simulink model "SPGF_FSK_0000_R2022b"  (R2022b)
settings: Solver=ode4  StartTime=0.0  StopTime=1.4  FixedStep=50e-6/50  RelTol=1e-3  EnableMultiTasking=on
undefined symbols (not defined in the file): D11, Delta
libraries: spsSeriesRLCBranchLib x1646, spsGroundLib x360, spsStairGeneratorLib x147, spsIdealSwitchLib x145, spsCurrentMeasurementLib x145, spsUniversalBridgeLib x76, spsThreePhaseSeriesRLCLoadLib x57, simulink x45, spsBistableLib x36, spsSequenceAnalyzerLib x31, spsThreePhaseParallelRLCLoadLib x20, spsThreePhaseTransformerTwoWindingsLib x20
(part 34 of 40)

== system SPGF_FSK_0000_R2022b/W60/Pi ==
  Ground{,1..8} (9 alike) : spsGroundLib/Ground  LConnTagsString=a
  Series RLC Branch{,1..2,27..28,33} (6 alike) : spsSeriesRLCBranchLib/Series RLC Branch  LConnTagsString=__new0  RConnTagsString=__new0  BranchType=RL  Resistance=R/2  Inductance=L/2  SetiL0=off  InitialCurrent=0  Capacitance=1e-6  Setx0=off  InitialVoltage=0  Measurements=None
  Series RLC Branch{10..11,13,29..30,32} (6 alike) : spsSeriesRLCBranchLib/Series RLC Branch  LConnTagsString=__new0  RConnTagsString=__new0  BranchType=R  Resistance=Rfg*4  Inductance=L/2  SetiL0=off  InitialCurrent=0  Capacitance=1e-6  Setx0=off  InitialVoltage=0  Measurements=None
  Series RLC Branch{9,12,14,31,40..41} (6 alike) : spsSeriesRLCBranchLib/Series RLC Branch  LConnTagsString=__new0  RConnTagsString=__new0  BranchType=C  Resistance=R/2  Inductance=L/2  SetiL0=off  InitialCurrent=0  Capacitance=Cfg*0.25  Setx0=off  InitialVoltage=0  Measurements=None
  Series RLC Branch15 : spsSeriesRLCBranchLib/Series RLC Branch  LConnTagsString=__new0  RConnTagsString=__new0  BranchType=R  Resistance=Rfg*2  Inductance=L/2  SetiL0=off  InitialCurrent=0  Capacitance=1e-6  Setx0=off  InitialVoltage=0  Measurements=None
  Series RLC Branch16 : spsSeriesRLCBranchLib/Series RLC Branch  LConnTagsString=__new0  RConnTagsString=__new0  BranchType=R  Resistance=Rfg*2  Inductance=L/2  SetiL0=off  InitialCurrent=0  Capacitance=1e-6  Setx0=off  InitialVoltage=0  Measurements=None
  Series RLC Branch17 : spsSeriesRLCBranchLib/Series RLC Branch  LConnTagsString=__new0  RConnTagsString=__new0  BranchType=C  Resistance=R/2  Inductance=L/2  SetiL0=off  InitialCurrent=0  Capacitance=Cfg*0.5  Setx0=off  InitialVoltage=0  Measurements=None
  Series RLC Branch18 : spsSeriesRLCBranchLib/Series RLC Branch  LConnTagsString=__new0  RConnTagsString=__new0  BranchType=R  Resistance=Rfg*2  Inductance=L/2  SetiL0=off  InitialCurrent=0  Capacitance=1e-6  Setx0=off  InitialVoltage=0  Measurements=None
  Series RLC Branch19 : spsSeriesRLCBranchLib/Series RLC Branch  LConnTagsString=__new0  RConnTagsString=__new0  BranchType=C  Resistance=R/2  Inductance=L/2  SetiL0=off  InitialCurrent=0  Capacitance=Cfg*0.5  Setx0=off  InitialVoltage=0  Measurements=None
  Series RLC Branch20 : spsSeriesRLCBranchLib/Series RLC Branch  LConnTagsString=__new0  RConnTagsString=__new0  BranchType=C  Resistance=R/2  Inductance=L/2  SetiL0=off  InitialCurrent=0  Capacitance=Cmf*0.5  Setx0=off  InitialVoltage=0  Measurements=None
  Series RLC Branch21 : spsSeriesRLCBranchLib/Series RLC Branch  LConnTagsString=__new0  RConnTagsString=__new0  BranchType=R  Resistance=Rmf*2  Inductance=L/2  SetiL0=off  InitialCurrent=0  Capacitance=1e-6  Setx0=off  InitialVoltage=0  Measurements=None
  Series RLC Branch22 : spsSeriesRLCBranchLib/Series RLC Branch  LConnTagsString=__new0  RConnTagsString=__new0  BranchType=C  Resistance=R/2  Inductance=L/2  SetiL0=off  InitialCurrent=0  Capacitance=Cmf*0.5  Setx0=off  InitialVoltage=0  Measurements=None
  Series RLC Branch23 : spsSeriesRLCBranchLib/Series RLC Branch  LConnTagsString=__new0  RConnTagsString=__new0  BranchType=R  Resistance=Rmf*2  Inductance=L/2  SetiL0=off  InitialCurrent=0  Capacitance=1e-6  Setx0=off  InitialVoltage=0  Measurements=None
  Series RLC Branch24 : spsSeriesRLCBranchLib/Series RLC Branch  LConnTagsString=__new0  RConnTagsString=__new0  BranchType=C  Resistance=R/2  Inductance=L/2  SetiL0=off  InitialCurrent=0  Capacitance=Cmf*0.5  Setx0=off  InitialVoltage=0  Measurements=None
  Series RLC Branch25 : spsSeriesRLCBranchLib/Series RLC Branch  LConnTagsString=__new0  RConnTagsString=__new0  BranchType=R  Resistance=Rmf*2  Inductance=L/2  SetiL0=off  InitialCurrent=0  Capacitance=1e-6  Setx0=off  InitialVoltage=0  Measurements=None
  Series RLC Branch26 : spsSeriesRLCBranchLib/Series RLC Branch  LConnTagsString=__new0  RConnTagsString=__new0  BranchType=C  Resistance=R/2  Inductance=L/2  SetiL0=off  InitialCurrent=0  Capacitance=Cfg*0.5  Setx0=off  InitialVoltage=0  Measurements=None
  Series RLC Branch{3,5,7,34,36,38} (6 alike) : spsSeriesRLCBranchLib/Series RLC Branch  LConnTagsString=__new0  RConnTagsString=__new0  BranchType=C  Resistance=R/2  Inductance=L/2  SetiL0=off  InitialCurrent=0  Capacitance=Cmf*0.25  Setx0=off  InitialVoltage=0  Measurements=None
  Series RLC Branch{4,6,8,35,37,39} (6 alike) : spsSeriesRLCBranchLib/Series RLC Branch  LConnTagsString=__new0  RConnTagsString=__new0  BranchType=R  Resistance=Rmf*4  Inductance=L/2  SetiL0=off  InitialCurrent=0  Capacitance=1e-6  Setx0=off  InitialVoltage=0  Measurements=None
  A : PMIOPort  Side=Left
  B : PMIOPort  Port=2  Side=Left
  C : PMIOPort  Port=3  Side=Left
  a : PMIOPort  Port=4  Side=Right
  b : PMIOPort  Port=5  Side=Right
  c : PMIOPort  Port=6  Side=Right
  connections:
  Series RLC Branch12/LConn1 -- Series RLC Branch11/LConn1 -- Series RLC Branch5/LConn1 -- Series RLC Branch6/LConn1 -- B/RConn1 -- Series RLC Branch4/RConn1 -- Series RLC Branch3/RConn1 -- Series RLC Branch1/LConn1
  Series RLC Branch13/LConn1 -- A/RConn1 -- Series RLC Branch4/LConn1 -- Series RLC Branch3/LConn1 -- Series RLC Branch7/LConn1 -- Series RLC Branch8/LConn1 -- Series RLC Branch/LConn1 -- Series RLC Branch14/LConn1
  Series RLC Branch9/LConn1 -- Series RLC Branch2/LConn1 -- Series RLC Branch8/RConn1 -- Series RLC Branch7/RConn1 -- C/RConn1 -- Series RLC Branch5/RConn1 -- Series RLC Branch6/RConn1 -- Series RLC Branch10/LConn1
  Series RLC Branch9/RConn1 -- Ground/LConn1 -- Series RLC Branch10/RConn1
  Series RLC Branch12/RConn1 -- Series RLC Branch11/RConn1 -- Ground1/LConn1
  Series RLC Branch13/RConn1 -- Series RLC Branch14/RConn1 -- Ground2/LConn1
  Series RLC Branch17/LConn1 -- Series RLC Branch16/LConn1 -- Series RLC Branch28/LConn1 -- Series RLC Branch1/RConn1 -- Series RLC Branch23/LConn1 -- Series RLC Branch22/LConn1 -- Series RLC Branch20/RConn1 -- Series RLC Branch21/RConn1
  Series RLC Branch21/LConn1 -- Series RLC Branch20/LConn1 -- Series RLC Branch/RConn1 -- Series RLC Branch27/LConn1 -- Series RLC Branch19/LConn1 -- Series RLC Branch18/LConn1 -- Series RLC Branch24/LConn1 -- Series RLC Branch25/LConn1
  Series RLC Branch26/LConn1 -- Series RLC Branch15/LConn1 -- Series RLC Branch2/RConn1 -- Series RLC Branch33/LConn1 -- Series RLC Branch25/RConn1 -- Series RLC Branch24/RConn1 -- Series RLC Branch22/RConn1 -- Series RLC Branch23/RConn1
  Series RLC Branch26/RConn1 -- Series RLC Branch15/RConn1 -- Ground3/LConn1
  Ground4/LConn1 -- Series RLC Branch17/RConn1 -- Series RLC Branch16/RConn1
  Ground5/LConn1 -- Series RLC Branch18/RConn1 -- Series RLC Branch19/RConn1
  Series RLC Branch31/LConn1 -- b/RConn1 -- Series RLC Branch35/RConn1 -- Series RLC Branch34/RConn1 -- Series RLC Branch36/LConn1 -- Series RLC Branch37/LConn1 -- Series RLC Branch28/RConn1 -- Series RLC Branch30/LConn1
  Series RLC Branch34/LConn1 -- a/RConn1 -- Series RLC Branch41/LConn1 -- Series RLC Branch32/LConn1 -- Series RLC Branch38/LConn1 -- Series RLC Branch39/LConn1 -- Series RLC Branch27/RConn1 -- Series RLC Branch35/LConn1
  Series RLC Branch29/LConn1 -- Series RLC Branch36/RConn1 -- Series RLC Branch37/RConn1 -- c/RConn1 -- Series RLC Branch39/RConn1 -- Series RLC Branch38/RConn1 -- Series RLC Branch33/RConn1 -- Series RLC Branch40/LConn1
  Series RLC Branch29/RConn1 -- Series RLC Branch40/RConn1 -- Ground6/LConn1
  Series RLC Branch31/RConn1 -- Series RLC Branch30/RConn1 -- Ground7/LConn1
  Series RLC Branch32/RConn1 -- Series RLC Branch41/RConn1 -- Ground8/LConn1

== system SPGF_FSK_0000_R2022b/W60/Q ==
  breaker : Subsystem  Commented=on  mask{SwitchA=off, SwitchB=off, SwitchC=off, InitialStatus=[1 1 1], BreakerResistance=0.0001, SnubberResistance=1e6, SnubberCapacitance=inf, TransitionTimes=[0.5 0.7], ShiftTimes=[0 0 0]}
      mask prompts: SwitchA "Switching of phase A"; SwitchB "Switching of phase B"; SwitchC "Switching of phase C"; InitialStatus "Initial status of phase breaker [A, B, C]"; BreakerResistance "Breaker resistance Ron (ohms) :"; SnubberResistance "Snubbers resistance Rp (ohms) :"; SnubberCapacitance "Snubbers capacitance Cp (F) :"; TransitionTimes "Transition times (s) :"; ShiftTimes "Time differences for switch [tA, tB, tC] (s) :"
      mask init: same as SPGF_FSK_0000_R2022b/Feed/Q/breaker
      mask Display:
      | % port_label('input',1,'Iabc');
      | 
      | port_label('lconn',1,'A');
      | port_label('lconn',2,'B');
      | port_label('lconn',3,'C');
      | 
      | port_label('rconn',1,'a');
      | port_label('rconn',2,'b');
      | port_label('rconn',3,'c');
      | 
      | disp('   Q    ');
  meas : Subsystem
  shunt : Subsystem
  A : PMIOPort  Side=Right
  B : PMIOPort  Port=2  Side=Right
  C : PMIOPort  Port=3  Side=Right
  a : PMIOPort  Port=4  Side=Left
  b : PMIOPort  Port=5  Side=Left
  c : PMIOPort  Port=6  Side=Left
  connections:
  shunt/LConn3 -- C/RConn1 -- breaker/LConn3
  shunt/LConn2 -- B/RConn1 -- breaker/LConn2
  A/RConn1 -- shunt/LConn1 -- breaker/LConn1
  meas/RConn1 -- a/RConn1
  meas/RConn2 -- b/RConn1
  meas/RConn3 -- c/RConn1
  meas/LConn3 -- breaker/RConn3 -- shunt/RConn3
  meas/LConn2 -- breaker/RConn2 -- shunt/RConn2
  meas/LConn1 -- breaker/RConn1 -- shunt/RConn1

== system SPGF_FSK_0000_R2022b/W60/concentrated ==
  Ccs/1 : spsSeriesRLCBranchLib/Series RLC Branch  LConnTagsString=__new0  RConnTagsString=__new0  BranchType=C  Resistance=190  Inductance=1e-3  SetiL0=off  InitialCurrent=0  Capacitance=-C_matrix(1,2)/2  Setx0=off  InitialVoltage=0  Measurements=None
  Ccs/2 : spsSeriesRLCBranchLib/Series RLC Branch  LConnTagsString=__new0  RConnTagsString=__new0  BranchType=C  Resistance=190  Inductance=1e-3  SetiL0=off  InitialCurrent=0  Capacitance=-C_matrix(1,2)/2  Setx0=off  InitialVoltage=0  Measurements=None
  Ccs2/1 : spsSeriesRLCBranchLib/Series RLC Branch  LConnTagsString=__new0  RConnTagsString=__new0  BranchType=C  Resistance=190  Inductance=1e-3  SetiL0=off  InitialCurrent=0  Capacitance=-C_matrix(3,4)/2  Setx0=off  InitialVoltage=0  Measurements=None
  Ccs2/2 : spsSeriesRLCBranchLib/Series RLC Branch  LConnTagsString=__new0  RConnTagsString=__new0  BranchType=C  Resistance=190  Inductance=1e-3  SetiL0=off  InitialCurrent=0  Capacitance=-C_matrix(3,4)/2  Setx0=off  InitialVoltage=0  Measurements=None
  Ccs2/3 : spsSeriesRLCBranchLib/Series RLC Branch  LConnTagsString=__new0  RConnTagsString=__new0  BranchType=R  Resistance=-Rg_matrix(3,4)*2  Inductance=1e-3  SetiL0=off  InitialCurrent=0  Capacitance=Rg_matrix(3,4)*2  Setx0=off  InitialVoltage=0  Measurements=None
  Ccs2/4 : spsSeriesRLCBranchLib/Series RLC Branch  LConnTagsString=__new0  RConnTagsString=__new0  BranchType=R  Resistance=-Rg_matrix(3,4)*2  Inductance=1e-3  SetiL0=off  InitialCurrent=0  Capacitance=Rg_matrix(3,4)*2  Setx0=off  InitialVoltage=0  Measurements=None
  Ccs3/1 : spsSeriesRLCBranchLib/Series RLC Branch  LConnTagsString=__new0  RConnTagsString=__new0  BranchType=C  Resistance=190  Inductance=1e-3  SetiL0=off  InitialCurrent=0  Capacitance=-C_matrix(5,6)/2  Setx0=off  InitialVoltage=0  Measurements=None
  Ccs3/2 : spsSeriesRLCBranchLib/Series RLC Branch  LConnTagsString=__new0  RConnTagsString=__new0  BranchType=C  Resistance=190  Inductance=1e-3  SetiL0=off  InitialCurrent=0  Capacitance=-C_matrix(5,6)/2  Setx0=off  InitialVoltage=0  Measurements=None
  Ccs3/3 : spsSeriesRLCBranchLib/Series RLC Branch  LConnTagsString=__new0  RConnTagsString=__new0  BranchType=R  Resistance=-Rg_matrix(5,6)*2  Inductance=1e-3  SetiL0=off  InitialCurrent=0  Capacitance=-C_matrix(5,6)/2  Setx0=off  InitialVoltage=0  Measurements=None
  Ccs3/4 : spsSeriesRLCBranchLib/Series RLC Branch  LConnTagsString=__new0  RConnTagsString=__new0  BranchType=R  Resistance=-Rg_matrix(5,6)*2  Inductance=1e-3  SetiL0=off  InitialCurrent=0  Capacitance=-C_matrix(5,6)/2  Setx0=off  InitialVoltage=0  Measurements=None
  Csg/2 : spsSeriesRLCBranchLib/Series RLC Branch  LConnTagsString=__new0  RConnTagsString=__new0  BranchType=C  Resistance=190  Inductance=1e-3  SetiL0=off  InitialCurrent=0  Capacitance=( C_matrix(1,2) + C_matrix(2,2) )/2  Setx0=off  InitialVoltage=0  Measurements=None
  Csg1/1 : spsSeriesRLCBranchLib/Series RLC Branch  LConnTagsString=__new0  RConnTagsString=__new0  BranchType=C  Resistance=190  Inductance=1e-3  SetiL0=off  InitialCurrent=0  Capacitance=( C_matrix(1,2) + C_matrix(2,2) )/2  Setx0=off  InitialVoltage=0  Measurements=None
  Csg2/1 : spsSeriesRLCBranchLib/Series RLC Branch  LConnTagsString=__new0  RConnTagsString=__new0  BranchType=C  Resistance=190  Inductance=1e-3  SetiL0=off  InitialCurrent=0  Capacitance=( C_matrix(3,4) + C_matrix(4,4) )/2  Setx0=off  InitialVoltage=0  Measurements=None
  Csg2/2 : spsSeriesRLCBranchLib/Series RLC Branch  LConnTagsString=__new0  RConnTagsString=__new0  BranchType=C  Resistance=190  Inductance=1e-3  SetiL0=off  InitialCurrent=0  Capacitance=( C_matrix(3,4) + C_matrix(4,4) )/2  Setx0=off  InitialVoltage=0  Measurements=None
  Csg3/1 : spsSeriesRLCBranchLib/Series RLC Branch  LConnTagsString=__new0  RConnTagsString=__new0  BranchType=C  Resistance=190  Inductance=1e-3  SetiL0=off  InitialCurrent=0  Capacitance=( C_matrix(5,6) + C_matrix(6,6) ) /2  Setx0=off  InitialVoltage=0  Measurements=None
  Csg3/2 : spsSeriesRLCBranchLib/Series RLC Branch  LConnTagsString=__new0  RConnTagsString=__new0  BranchType=C  Resistance=190  Inductance=1e-3  SetiL0=off  InitialCurrent=0  Capacitance=( C_matrix(5,6) + C_matrix(6,6) ) /2  Setx0=off  InitialVoltage=0  Measurements=None
  Ground{1..4} (4 alike) : spsGroundLib/Ground  LConnTagsString=a
  RL : spsMutualInductanceLib/Mutual Inductance  LConnTagsString=a|b|c|L4|L5|L6  RConnTagsString=A|B|C|R4|R5|R6  TypeOfMutual=Generalized mutual inductance  NumberOfWindings=6  SelfImpedance1=[1.1 1.1e-03]  SelfImpedance2=[ 1.1 1.1e-03]  ThreeWindings=on  SelfImpedance3=[ 1.1 1.1e-03]  MutualImpedance=[1.0 1.0e-03]  InductanceMatrix=L_matrix  ResistanceMatrix=R_matrix  Measurements=None
      settings: LibrarySourceBlock=sps_lib/Passives/Mutual Inductance
  Rcs*2 : spsSeriesRLCBranchLib/Series RLC Branch  LConnTagsString=__new0  RConnTagsString=__new0  BranchType=R  Resistance=-Rg_matrix(1,2)*2  Inductance=1e-3  SetiL0=off  InitialCurrent=0  Capacitance=Rg_matrix(1,2)*2  Setx0=off  InitialVoltage=0  Measurements=None
  Rgcs1/1 : spsSeriesRLCBranchLib/Series RLC Branch  LConnTagsString=__new0  RConnTagsString=__new0  BranchType=R  Resistance=-Rg_matrix(1,2)*2  Inductance=1e-3  SetiL0=off  InitialCurrent=0  Capacitance=Rg_matrix(1,2)*2  Setx0=off  InitialVoltage=0  Measurements=None
  Rgsg1/1 : spsSeriesRLCBranchLib/Series RLC Branch  LConnTagsString=__new0  RConnTagsString=__new0  BranchType=R  Resistance=(Rg_matrix(4,4)+Rg_matrix(3,4))*2  Inductance=1e-3  SetiL0=off  InitialCurrent=0  Capacitance=Rg_matrix(1,2)*2  Setx0=off  InitialVoltage=0  Measurements=None
  Rgsg1/2 : spsSeriesRLCBranchLib/Series RLC Branch  LConnTagsString=__new0  RConnTagsString=__new0  BranchType=R  Resistance=(Rg_matrix(2,2)+Rg_matrix(1,2))*2  Inductance=1e-3  SetiL0=off  InitialCurrent=0  Capacitance=Rg_matrix(1,2)*2  Setx0=off  InitialVoltage=0  Measurements=None
  Rgsg1/3 : spsSeriesRLCBranchLib/Series RLC Branch  LConnTagsString=__new0  RConnTagsString=__new0  BranchType=R  Resistance=(Rg_matrix(4,4)+Rg_matrix(3,4))*2  Inductance=1e-3  SetiL0=off  InitialCurrent=0  Capacitance=Rg_matrix(1,2)*2  Setx0=off  InitialVoltage=0  Measurements=None
  Rgsg1/4 : spsSeriesRLCBranchLib/Series RLC Branch  LConnTagsString=__new0  RConnTagsString=__new0  BranchType=R  Resistance=(Rg_matrix(2,2)+Rg_matrix(1,2))*2  Inductance=1e-3  SetiL0=off  InitialCurrent=0  Capacitance=Rg_matrix(1,2)*2  Setx0=off  InitialVoltage=0  Measurements=None
  Rsg*2 : spsSeriesRLCBranchLib/Series RLC Branch  LConnTagsString=__new0  RConnTagsString=__new0  BranchType=R  Resistance=(Rg_matrix(6,6)+Rg_matrix(5,6))*2  Inductance=1e-3  SetiL0=off  InitialCurrent=0  Capacitance=Rg_matrix(1,2)*2  Setx0=off  InitialVoltage=0  Measurements=None
  Rsg1/1 : spsSeriesRLCBranchLib/Series RLC Branch  LConnTagsString=__new0  RConnTagsString=__new0  BranchType=R  Resistance=(Rg_matrix(6,6)+Rg_matrix(5,6))*2  Inductance=1e-3  SetiL0=off  InitialCurrent=0  Capacitance=Rg_matrix(1,2)*2  Setx0=off  InitialVoltage=0  Measurements=None
  A : PMIOPort  Side=Left
  B : PMIOPort  Port=2  Side=Left
  C : PMIOPort  Port=3  Side=Left
  a : PMIOPort  Port=4  Side=Right
  b : PMIOPort  Port=5  Side=Right
  c : PMIOPort  Port=6  Side=Right
  connections:
  RL/LConn6 -- Ground3/LConn1 -- Rgsg1/2/LConn1 -- Csg/2/LConn1 -- Rcs*2/LConn1 -- Ccs/2/LConn1 -- RL/LConn2 -- RL/LConn4 -- Rgsg1/1/LConn1 -- Csg2/2/LConn1 -- Ccs2/3/LConn1 -- Ccs2/2/LConn1 -- Rsg*2/LConn1 -- Csg3/2/LConn1 -- Ccs3/3/LConn1 -- Ccs3/2/LConn1
  Rsg1/1/RConn1 -- Rgsg1/3/RConn1 -- Rgsg1/4/RConn1 -- Csg3/1/RConn1 -- Csg2/1/RConn1 -- Ground2/LConn1 -- Csg1/1/RConn1
  Rgsg1/3/LConn1 -- Ccs2/4/LConn1 -- Csg2/1/LConn1 -- Ccs2/1/LConn1 -- RL/RConn4 -- Rgsg1/4/LConn1 -- Rgcs1/1/LConn1 -- Csg1/1/LConn1 -- Ccs/1/LConn1 -- RL/RConn2 -- Ground4/LConn1 -- RL/RConn6 -- Ccs3/1/LConn1 -- Rsg1/1/LConn1 -- Ccs3/4/LConn1 -- Csg3/1/LConn1
  Rsg*2/RConn1 -- Rgsg1/1/RConn1 -- Rgsg1/2/RConn1 -- Csg3/2/RConn1 -- Csg2/2/RConn1 -- Ground1/LConn1 -- Csg/2/RConn1
  a/RConn1 -- RL/RConn1 -- Rgcs1/1/RConn1 -- Ccs/1/RConn1
  b/RConn1 -- RL/RConn3 -- Ccs2/4/RConn1 -- Ccs2/1/RConn1
  Ccs3/1/RConn1 -- c/RConn1 -- RL/RConn5 -- Ccs3/4/RConn1
  RL/LConn1 -- A/RConn1 -- Rcs*2/RConn1 -- Ccs/2/RConn1
  RL/LConn3 -- B/RConn1 -- Ccs2/3/RConn1 -- Ccs2/2/RConn1
  Ccs3/2/RConn1 -- C/RConn1 -- RL/LConn5 -- Ccs3/3/RConn1

== system SPGF_FSK_0000_R2022b/W61/Q ==
  breaker : Subsystem  Commented=on  mask{SwitchA=off, SwitchB=off, SwitchC=off, InitialStatus=[1 1 1], BreakerResistance=0.0001, SnubberResistance=1e6, SnubberCapacitance=inf, TransitionTimes=[0.5 0.7], ShiftTimes=[0 0 0]}
      mask prompts: SwitchA "Switching of phase A"; SwitchB "Switching of phase B"; SwitchC "Switching of phase C"; InitialStatus "Initial status of phase breaker [A, B, C]"; BreakerResistance "Breaker resistance Ron (ohms) :"; SnubberResistance "Snubbers resistance Rp (ohms) :"; SnubberCapacitance "Snubbers capacitance Cp (F) :"; TransitionTimes "Transition times (s) :"; ShiftTimes "Time differences for switch [tA, tB, tC] (s) :"
      mask init: same as SPGF_FSK_0000_R2022b/Feed/Q/breaker
      mask Display:
      | % port_label('input',1,'Iabc');
      | 
      | port_label('lconn',1,'A');
      | port_label('lconn',2,'B');
      | port_label('lconn',3,'C');
      | 
      | port_label('rconn',1,'a');
      | port_label('rconn',2,'b');
      | port_label('rconn',3,'c');
      | 
      | disp('   Q    ');
  meas : Subsystem
  shunt : Subsystem
  A : PMIOPort  Side=Right
  B : PMIOPort  Port=2  Side=Right
  C : PMIOPort  Port=3  Side=Right
  a : PMIOPort  Port=4  Side=Left
  b : PMIOPort  Port=5  Side=Left
  c : PMIOPort  Port=6  Side=Left
  connections:
  shunt/RConn1 -- breaker/RConn1 -- meas/LConn1
  shunt/RConn2 -- breaker/RConn2 -- meas/LConn2
  shunt/RConn3 -- breaker/RConn3 -- meas/LConn3
  meas/RConn3 -- c/RConn1
  meas/RConn2 -- b/RConn1
  meas/RConn1 -- a/RConn1
  breaker/LConn1 -- shunt/LConn1 -- A/RConn1
  breaker/LConn2 -- B/RConn1 -- shunt/LConn2
  breaker/LConn3 -- C/RConn1 -- shunt/LConn3

== system SPGF_FSK_0000_R2022b/measurements/Fourier Block abc ==
  abc : Inport
  Demux1 : Demux  Commented=on  Outputs=9
  Scope13 : Scope
  Sequence Analyzer9 : spsSequenceAnalyzerLib/Sequence Analyzer  Freq=50  n=17  seq=Positive  InInit=[0, 0]  Ts=FTime
      settings: LibrarySourceBlock=sps_lib/Sensors and Measurements/Sequence Analyzer
  Terminator9 : Terminator
  wires:
  abc/1 -> Sequence Analyzer9/1
  Sequence Analyzer9/2 -> Terminator9/1
  Sequence Analyzer9/1 -> Scope13/1, Demux1/1

== system SPGF_FSK_0000_R2022b/measurements/Fourier Block u ==
  u : Inport
  Demux1 : Demux  Commented=on  Outputs=9
  Fourier10 : spsFourierLib/Fourier  Freq=50  n=[1 2 3 5 7 9 11 13 17]  InInit=[0, 0]  Ts=FTime
  Scope13 : Scope
  Terminator10 : Terminator
  wires:
  u/1 -> Fourier10/1
  Fourier10/1 -> Demux1/1, Scope13/1
  Fourier10/2 -> Terminator10/1

== system SPGF_FSK_0000_R2022b/measurements/PQ1 ==
  Vmag_seq : Inport
  Vang : Inport  Port=2
  Imag_seq : Inport  Port=3
  Iang : Inport  Port=4
  Deg->Rad : Gain  Gain=pi/180  SaturateOnIntegerOverflow=on  OutDataTypeStr=Inherit: Same as input  ParamDataTypeStr=Inherit: Same as input
  Gain1 : Gain  Gain=3/2  SaturateOnIntegerOverflow=on  OutDataTypeStr=Inherit: Same as input  ParamDataTypeStr=Inherit: Same as input
  Product : Product  InputSameDT=on  SaturateOnIntegerOverflow=on  OutDataTypeStr=Inherit: Same as first input
  Product1 : Product  InputSameDT=on  SaturateOnIntegerOverflow=on  OutDataTypeStr=Inherit: Same as first input
  Product3 : Product  InputSameDT=on  SaturateOnIntegerOverflow=on  OutDataTypeStr=Inherit: Same as first input
  Sum : Sum  Inputs=+-  InputSameDT=on  SaturateOnIntegerOverflow=on  OutDataTypeStr=Inherit: Same as first input
  Trigonometric Function1 : Trigonometry  Operator=cos
  Trigonometric Function2 : Trigonometry
  P : Outport
  Q : Outport  Port=2
  wires:
  Trigonometric Function1/1 -> Product1/2
  Sum/1 -> Deg->Rad/1
  Imag_seq/1 -> Product/2
  Product/1 -> Gain1/1  "V1 *I1"
  Trigonometric Function2/1 -> Product3/2
  Gain1/1 -> Product1/1, Product3/1
  Vmag_seq/1 -> Product/1
  Deg->Rad/1 -> Trigonometric Function2/1, Trigonometric Function1/1  "phi"
  Product3/1 -> Q/1
  Iang/1 -> Sum/2
  Vang/1 -> Sum/1
  Product1/1 -> P/1

== system SPGF_FSK_0000_R2022b/measurements/PQ8 ==
  Vmag_seq : Inport
  Vang : Inport  Port=2
  Imag_seq : Inport  Port=3
  Iang : Inport  Port=4
  Deg->Rad : Gain  Gain=pi/180  SaturateOnIntegerOverflow=on  OutDataTypeStr=Inherit: Same as input  ParamDataTypeStr=Inherit: Same as input
  Gain1 : Gain  Gain=3/2  SaturateOnIntegerOverflow=on  OutDataTypeStr=Inherit: Same as input  ParamDataTypeStr=Inherit: Same as input
  Product : Product  InputSameDT=on  SaturateOnIntegerOverflow=on  OutDataTypeStr=Inherit: Same as first input
  Product1 : Product  InputSameDT=on  SaturateOnIntegerOverflow=on  OutDataTypeStr=Inherit: Same as first input
  Product3 : Product  InputSameDT=on  SaturateOnIntegerOverflow=on  OutDataTypeStr=Inherit: Same as first input
  Sum : Sum  Inputs=+-  InputSameDT=on  SaturateOnIntegerOverflow=on  OutDataTypeStr=Inherit: Same as first input
  Trigonometric Function1 : Trigonometry  Operator=cos
  Trigonometric Function2 : Trigonometry
  P : Outport
  Q : Outport  Port=2
  wires:
  Product1/1 -> P/1
  Vang/1 -> Sum/1
  Iang/1 -> Sum/2
  Product3/1 -> Q/1
  Deg->Rad/1 -> Trigonometric Function1/1, Trigonometric Function2/1  "phi"
  Vmag_seq/1 -> Product/1
  Gain1/1 -> Product3/1, Product1/1
  Trigonometric Function2/1 -> Product3/2
  Product/1 -> Gain1/1  "V1 *I1"
  Imag_seq/1 -> Product/2
  Sum/1 -> Deg->Rad/1
  Trigonometric Function1/1 -> Product1/2

== system SPGF_FSK_0000_R2022b/measurements/RMS1 ==
  abc : Inport
  Gain25 : Gain  Gain=1/sqrt(2)
  Rate Transition : RateTransition
  Rate Transition1 : RateTransition
  Sequence Analyzer : spsSequenceAnalyzerLib/Sequence Analyzer  Freq=50  n=1  seq=Positive  InInit=[1, 0]  Ts=FTime
      settings: LibrarySourceBlock=sps_lib/Sensors and Measurements/Sequence Analyzer
  Terminator19 : Terminator
  I1 : Outport
  wires:
  Sequence Analyzer/2 -> Terminator19/1
  Gain25/1 -> Rate Transition1/1
  Sequence Analyzer/1 -> Gain25/1
  abc/1 -> Rate Transition/1
  Rate Transition/1 -> Sequence Analyzer/1
  Rate Transition1/1 -> I1/1

== system SPGF_FSK_0000_R2022b/measurements/RMS10 ==
  i : Inport
  Fourier36 : spsFourierLib/Fourier  Freq=50  n=1  InInit=[0, 0]  Ts=FTime
  Gain25 : Gain  Gain=1/sqrt(2)
  Rate Transition : RateTransition
  Rate Transition1 : RateTransition
  Terminator19 : Terminator
  I : Outport
  wires:
  Rate Transition1/1 -> I/1
  Rate Transition/1 -> Fourier36/1
  Fourier36/2 -> Terminator19/1
  Gain25/1 -> Rate Transition1/1
  Fourier36/1 -> Gain25/1
  i/1 -> Rate Transition/1

== system SPGF_FSK_0000_R2022b/measurements/RMS11 ==
  i : Inport
  Fourier36 : spsFourierLib/Fourier  Freq=50  n=1  InInit=[0, 0]  Ts=FTime
  Gain25 : Gain  Gain=1/sqrt(2)
  Rate Transition : RateTransition
  Rate Transition1 : RateTransition
  Terminator19 : Terminator
  I : Outport
  wires:
  i/1 -> Rate Transition/1
  Fourier36/1 -> Gain25/1
  Gain25/1 -> Rate Transition1/1
  Fourier36/2 -> Terminator19/1
  Rate Transition/1 -> Fourier36/1
  Rate Transition1/1 -> I/1

== system SPGF_FSK_0000_R2022b/measurements/RMS12 ==
  abc : Inport
  Gain25 : Gain  Gain=1/sqrt(2)
  Rate Transition : RateTransition
  Rate Transition1 : RateTransition
  Sequence Analyzer : spsSequenceAnalyzerLib/Sequence Analyzer  Freq=50  n=1  seq=Positive  InInit=[1, 0]  Ts=FTime
      settings: LibrarySourceBlock=sps_lib/Sensors and Measurements/Sequence Analyzer
  Terminator19 : Terminator
  I1 : Outport
  wires:
  Sequence Analyzer/2 -> Terminator19/1
  Gain25/1 -> Rate Transition1/1
  Sequence Analyzer/1 -> Gain25/1
  abc/1 -> Rate Transition/1
  Rate Transition/1 -> Sequence Analyzer/1
  Rate Transition1/1 -> I1/1

== system SPGF_FSK_0000_R2022b/measurements/RMS13 ==
  i : Inport
  Fourier36 : spsFourierLib/Fourier  Freq=50  n=1  InInit=[0, 0]  Ts=FTime
  Gain25 : Gain  Gain=1/sqrt(2)
  Rate Transition : RateTransition
  Rate Transition1 : RateTransition
  Terminator19 : Terminator
  I : Outport
  wires:
  Rate Transition1/1 -> I/1
  Rate Transition/1 -> Fourier36/1
  Fourier36/2 -> Terminator19/1
  Gain25/1 -> Rate Transition1/1
  Fourier36/1 -> Gain25/1
  i/1 -> Rate Transition/1

== system SPGF_FSK_0000_R2022b/measurements/RMS14 ==
  abc : Inport
  Gain25 : Gain  Gain=1/sqrt(2)
  Rate Transition : RateTransition
  Rate Transition1 : RateTransition
  Sequence Analyzer : spsSequenceAnalyzerLib/Sequence Analyzer  Freq=50  n=1  seq=Positive  InInit=[1, 0]  Ts=FTime
      settings: LibrarySourceBlock=sps_lib/Sensors and Measurements/Sequence Analyzer
  Terminator19 : Terminator
  I1 : Outport
  wires:
  Rate Transition1/1 -> I1/1
  Rate Transition/1 -> Sequence Analyzer/1
  abc/1 -> Rate Transition/1
  Sequence Analyzer/1 -> Gain25/1
  Gain25/1 -> Rate Transition1/1
  Sequence Analyzer/2 -> Terminator19/1

== system SPGF_FSK_0000_R2022b/measurements/RMS2 ==
  i : Inport
  Fourier36 : spsFourierLib/Fourier  Freq=50  n=1  InInit=[0, 0]  Ts=FTime
  Gain25 : Gain  Gain=1/sqrt(2)
  Rate Transition : RateTransition
  Rate Transition1 : RateTransition
  Terminator19 : Terminator
  I : Outport
  wires:
  i/1 -> Rate Transition/1
  Fourier36/1 -> Gain25/1
  Gain25/1 -> Rate Transition1/1
  Fourier36/2 -> Terminator19/1
  Rate Transition/1 -> Fourier36/1
  Rate Transition1/1 -> I/1

== system SPGF_FSK_0000_R2022b/measurements/RMS3 ==
  abc : Inport
  Gain25 : Gain  Gain=1/sqrt(2)
  Rate Transition : RateTransition
  Rate Transition1 : RateTransition
  Sequence Analyzer : spsSequenceAnalyzerLib/Sequence Analyzer  Freq=50  n=1  seq=Positive  InInit=[1, 0]  Ts=FTime
      settings: LibrarySourceBlock=sps_lib/Sensors and Measurements/Sequence Analyzer
  Terminator19 : Terminator
  I1 : Outport
  wires:
  Rate Transition1/1 -> I1/1
  Rate Transition/1 -> Sequence Analyzer/1
  abc/1 -> Rate Transition/1
  Sequence Analyzer/1 -> Gain25/1
  Gain25/1 -> Rate Transition1/1
  Sequence Analyzer/2 -> Terminator19/1

== system SPGF_FSK_0000_R2022b/measurements/RMS36 ==
  abc : Inport
  Gain25 : Gain  Gain=1/sqrt(2)
  Sequence Analyzer : spsSequenceAnalyzerLib/Sequence Analyzer  Freq=50  n=1  seq=Positive  InInit=[1, 0]  Ts=FTime
      settings: LibrarySourceBlock=sps_lib/Sensors and Measurements/Sequence Analyzer
  Terminator19 : Terminator
  I1 : Outport
  wires:
  abc/1 -> Sequence Analyzer/1
  Sequence Analyzer/1 -> Gain25/1
  Gain25/1 -> I1/1
  Sequence Analyzer/2 -> Terminator19/1

== system SPGF_FSK_0000_R2022b/measurements/RMS4 ==
  i : Inport
  Fourier36 : spsFourierLib/Fourier  Freq=50  n=1  InInit=[0, 0]  Ts=FTime
  Gain25 : Gain  Gain=1/sqrt(2)
  Rate Transition : RateTransition
  Rate Transition1 : RateTransition
  Terminator19 : Terminator
  I : Outport
  wires:
  Rate Transition1/1 -> I/1
  Rate Transition/1 -> Fourier36/1
  Fourier36/2 -> Terminator19/1
  Gain25/1 -> Rate Transition1/1
  Fourier36/1 -> Gain25/1
  i/1 -> Rate Transition/1

== system SPGF_FSK_0000_R2022b/measurements/RMS44 ==
  abc : Inport
  Gain25 : Gain  Gain=1/sqrt(2)
  Sequence Analyzer : spsSequenceAnalyzerLib/Sequence Analyzer  Freq=50  n=1  seq=Positive  InInit=[1, 0]  Ts=FTime
      settings: LibrarySourceBlock=sps_lib/Sensors and Measurements/Sequence Analyzer
  Terminator19 : Terminator
  I1 : Outport
  wires:
  Sequence Analyzer/2 -> Terminator19/1
  Gain25/1 -> I1/1
  Sequence Analyzer/1 -> Gain25/1
  abc/1 -> Sequence Analyzer/1

== system SPGF_FSK_0000_R2022b/measurements/RMS45 ==
  abc : Inport
  Gain25 : Gain  Gain=1/sqrt(2)
  Sequence Analyzer : spsSequenceAnalyzerLib/Sequence Analyzer  Freq=50  n=1  seq=Positive  InInit=[1, 0]  Ts=FTime
      settings: LibrarySourceBlock=sps_lib/Sensors and Measurements/Sequence Analyzer
  Terminator19 : Terminator
  I1 : Outport
  wires:
  abc/1 -> Sequence Analyzer/1
  Sequence Analyzer/1 -> Gain25/1
  Gain25/1 -> I1/1
  Sequence Analyzer/2 -> Terminator19/1

== system SPGF_FSK_0000_R2022b/measurements/RMS46 ==
  i : Inport
  Fourier36 : spsFourierLib/Fourier  Freq=50  n=1  InInit=[0, 0]  Ts=FTime
  Gain25 : Gain  Gain=1/sqrt(2)
  Terminator19 : Terminator
  I : Outport
  wires:
  Fourier36/2 -> Terminator19/1
  Gain25/1 -> I/1
  Fourier36/1 -> Gain25/1
  i/1 -> Fourier36/1

== system SPGF_FSK_0000_R2022b/measurements/RMS5 ==
  abc : Inport
  Gain25 : Gain  Gain=1/sqrt(2)
  Rate Transition : RateTransition
  Rate Transition1 : RateTransition
  Sequence Analyzer : spsSequenceAnalyzerLib/Sequence Analyzer  Freq=50  n=1  seq=Positive  InInit=[1, 0]  Ts=FTime
      settings: LibrarySourceBlock=sps_lib/Sensors and Measurements/Sequence Analyzer
  Terminator19 : Terminator
  I1 : Outport
  wires:
  Rate Transition1/1 -> I1/1
  Rate Transition/1 -> Sequence Analyzer/1
  abc/1 -> Rate Transition/1
  Sequence Analyzer/1 -> Gain25/1
  Gain25/1 -> Rate Transition1/1
  Sequence Analyzer/2 -> Terminator19/1

== system SPGF_FSK_0000_R2022b/measurements/RMS6 ==
  i : Inport
  Fourier36 : spsFourierLib/Fourier  Freq=50  n=1  InInit=[0, 0]  Ts=FTime
  Gain25 : Gain  Gain=1/sqrt(2)
  Rate Transition : RateTransition
  Rate Transition1 : RateTransition
  Terminator19 : Terminator
  I : Outport
  wires:
  Rate Transition1/1 -> I/1
  Rate Transition/1 -> Fourier36/1
  Fourier36/2 -> Terminator19/1
  Gain25/1 -> Rate Transition1/1
  Fourier36/1 -> Gain25/1
  i/1 -> Rate Transition/1

== system SPGF_FSK_0000_R2022b/measurements/RMS7 ==
  abc : Inport
  Gain25 : Gain  Gain=1/sqrt(2)
  Rate Transition : RateTransition
  Rate Transition1 : RateTransition
  Sequence Analyzer : spsSequenceAnalyzerLib/Sequence Analyzer  Freq=50  n=1  seq=Positive  InInit=[1, 0]  Ts=FTime
      settings: LibrarySourceBlock=sps_lib/Sensors and Measurements/Sequence Analyzer
  Terminator19 : Terminator
  I1 : Outport
  wires:
  Sequence Analyzer/2 -> Terminator19/1
  Gain25/1 -> Rate Transition1/1
  Sequence Analyzer/1 -> Gain25/1
  abc/1 -> Rate Transition/1
  Rate Transition/1 -> Sequence Analyzer/1
  Rate Transition1/1 -> I1/1

== system SPGF_FSK_0000_R2022b/measurements/RMS8 ==
  i : Inport
  Fourier36 : spsFourierLib/Fourier  Freq=50  n=1  InInit=[0, 0]  Ts=FTime
  Gain25 : Gain  Gain=1/sqrt(2)
  Rate Transition : RateTransition
  Rate Transition1 : RateTransition
  Terminator19 : Terminator
  I : Outport
  wires:
  i/1 -> Rate Transition/1
  Fourier36/1 -> Gain25/1
  Gain25/1 -> Rate Transition1/1
  Fourier36/2 -> Terminator19/1
  Rate Transition/1 -> Fourier36/1
  Rate Transition1/1 -> I/1

== system SPGF_FSK_0000_R2022b/measurements/RMS9 ==
  abc : Inport
  Gain25 : Gain  Gain=1/sqrt(2)
  Rate Transition : RateTransition
  Rate Transition1 : RateTransition
  Sequence Analyzer : spsSequenceAnalyzerLib/Sequence Analyzer  Freq=50  n=1  seq=Positive  InInit=[1, 0]  Ts=FTime
      settings: LibrarySourceBlock=sps_lib/Sensors and Measurements/Sequence Analyzer
  Terminator19 : Terminator
  I1 : Outport
  wires:
  Rate Transition1/1 -> I1/1
  Rate Transition/1 -> Sequence Analyzer/1
  abc/1 -> Rate Transition/1
  Sequence Analyzer/1 -> Gain25/1
  Gain25/1 -> Rate Transition1/1
  Sequence Analyzer/2 -> Terminator19/1

== system SPGF_FSK_0000_R2022b/measurements/RXZ1 ==
  Vmag_seq : Inport
  Vang : Inport  Port=2
  Imag_seq : Inport  Port=3
  Iang : Inport  Port=4
  Add : Sum  Inputs=+-
  Divide : Product  Inputs=*/
  Gain : Gain  Gain=pi/180
  Product : Product
  Product1 : Product
  Trigonometric Function : Trigonometry
  Trigonometric Function1 : Trigonometry  Operator=cos
  R : Outport
  X : Outport  Port=2
  Z : Outport  Port=3
  Zang : Outport  Port=4
  wires:
  Iang/1 -> Add/2
  Trigonometric Function/1 -> Product1/2
  Trigonometric Function1/1 -> Product/2
  Vang/1 -> Add/1
  Divide/1 -> Z/1, Product/1, Product1/1
  Product1/1 -> X/1
  Product/1 -> R/1
  Imag_seq/1 -> Divide/2
  Vmag_seq/1 -> Divide/1
  Gain/1 -> Trigonometric Function/1, Trigonometric Function1/1
  Add/1 -> Zang/1, Gain/1

== system SPGF_FSK_0000_R2022b/measurements/RXZ7 ==
  Vmag_seq : Inport
  Vang : Inport  Port=2
  Imag_seq : Inport  Port=3
  Iang : Inport  Port=4
  Add : Sum  Inputs=+-
  Divide : Product  Inputs=*/
  Gain : Gain  Gain=pi/180
  Product : Product
  Product1 : Product
  Trigonometric Function : Trigonometry
  Trigonometric Function1 : Trigonometry  Operator=cos
  R : Outport
  X : Outport  Port=2
  Z : Outport  Port=3
  Zang : Outport  Port=4
  wires:
  Add/1 -> Gain/1, Zang/1
  Gain/1 -> Trigonometric Function1/1, Trigonometric Function/1
  Vmag_seq/1 -> Divide/1
  Imag_seq/1 -> Divide/2
  Product/1 -> R/1
  Product1/1 -> X/1
  Divide/1 -> Product1/1, Product/1, Z/1
  Vang/1 -> Add/1
  Trigonometric Function1/1 -> Product/2
  Trigonometric Function/1 -> Product1/2
  Iang/1 -> Add/2

== system SPGF_FSK_0000_R2022b/spgf/Control ==
  m : Inport
  Add : Sum  Inputs=+-
  Arcing : Subsystem  TreatAsAtomicUnit=on
  Count Limiter : Subsystem
  Ctrl : Product  Inputs=****
  Fault A2 : Constant  Value=LimitArcNum
  Fault A3 : Constant  Value=AddTimeDelay
  Fault A4 : Constant  Value=Inter
  InitialPhaseCtrl : Subsystem  TreatAsAtomicUnit=on
  Interruption : Subsystem
  One : Constant
  SW_Int : Switch  Criteria=u2 > Threshold  Threshold=0.5  SaturateOnIntegerOverflow=off  InputSameDT=off
  SW_Limit : Switch  Criteria=u2 > Threshold  Threshold=0.5  SaturateOnIntegerOverflow=off  InputSameDT=off
  SW_TD : Switch  Criteria=u2 > Threshold  Threshold=0.5  SaturateOnIntegerOverflow=off  InputSameDT=off
  Step : Step  Time=EndFaultTime  SampleTime=0
  Step1 : Step  Time=BeginFaultTime  SampleTime=0
  Time Delay : Subsystem
  g : Outport
  wires:
  Interruption/1(O) -> SW_Int/3, [Inter]
  [Inter] -> Arcing/2(Inter)
  Ctrl/1 -> Time Delay/2(Control), SW_TD/3
  InitialPhaseCtrl/1(O) -> Ctrl/3
  SW_TD/1 -> SW_Limit/3, Count Limiter/1(I)
  Step/1 -> Add/2
  Count Limiter/2(O) -> SW_Limit/1
  Fault A4/1 -> SW_Int/2
  [F] -> Arcing/Enable
  SW_Int/1 -> Ctrl/4
  [F] -> InitialPhaseCtrl/Enable
  Step1/1 -> Add/1
  m/1 -> Arcing/1(m), InitialPhaseCtrl/1(m)
  Add/1 -> [F], Ctrl/1
  Arcing/1(O) -> Ctrl/2
  Fault A2/1 -> SW_Limit/2
  Count Limiter/1(Count) -> Time Delay/1(Count)
  Time Delay/1(O) -> SW_TD/1
  Fault A3/1 -> SW_TD/2
  One/1 -> SW_Int/1
  SW_Limit/1 -> g/1

== system SPGF_FSK_0000_R2022b/Feed/Q/breaker ==
  Fault A2 : Constant  Value=InitialStatus(3)
  Fault A3 : Constant  Value=InitialStatus(2)
  Fault A4 : Constant  Value=InitialStatus(1)
  Fault C1 : Constant  Value=SwitchC
  Fault C2 : Constant  Value=SwitchB
  Fault C3 : Constant  Value=SwitchA
  Ideal Switch A : spsIdealSwitchLib/Ideal Switch  Ron=BreakerResistance  Lon=0  IC=InitialStatus(1)  Rs=SnubberResistance  Cs=SnubberCapacitance  Measurements=off
  Ideal Switch B : spsIdealSwitchLib/Ideal Switch  Ron=BreakerResistance  Lon=0  IC=InitialStatus(2)  Rs=SnubberResistance  Cs=SnubberCapacitance  Measurements=off
  Ideal Switch C : spsIdealSwitchLib/Ideal Switch  Ron=BreakerResistance  Lon=0  IC=InitialStatus(3)  Rs=SnubberResistance  Cs=SnubberCapacitance  Measurements=off
  Stair Generator A : spsStairGeneratorLib/Stair Generator  t=SwitchTimesA  e=SwitchStatusA  Ts=0
  Stair Generator B : spsStairGeneratorLib/Stair Generator  t=SwitchTimesB  e=SwitchStatusB  Ts=0
  Stair Generator C : spsStairGeneratorLib/Stair Generator  t=SwitchTimesB  e=SwitchStatusB  Ts=0
  Switch2 : Switch  Criteria=u2 > Threshold  Threshold=0.5  SaturateOnIntegerOverflow=off  InputSameDT=off
  Switch3 : Switch  Criteria=u2 > Threshold  Threshold=0.5  SaturateOnIntegerOverflow=off  InputSameDT=off
  Switch4 : Switch  Criteria=u2 > Threshold  Threshold=0.5  SaturateOnIntegerOverflow=off  InputSameDT=off
  A : PMIOPort  Side=Left
  B : PMIOPort  Port=2  Side=Left
  C : PMIOPort  Port=3  Side=Left
  a : PMIOPort  Port=4  Side=Right
  b : PMIOPort  Port=5  Side=Right
  c : PMIOPort  Port=6  Side=Right
  wires:
  Switch2/1 -> Ideal Switch C/1
  Fault A2/1 -> Switch2/3
  Fault C1/1 -> Switch2/2
  Switch3/1 -> Ideal Switch B/1
  Fault A3/1 -> Switch3/3
  Fault C2/1 -> Switch3/2
  Fault A4/1 -> Switch4/3
  Fault C3/1 -> Switch4/2
  Switch4/1 -> Ideal Switch A/1
  Stair Generator B/1 -> Switch3/1
  Stair Generator A/1 -> Switch4/1
  Stair Generator C/1 -> Switch2/1
  connections:
  Ideal Switch B/LConn1 -- B/RConn1
  Ideal Switch A/LConn1 -- A/RConn1
  Ideal Switch C/LConn1 -- C/RConn1
  Ideal Switch A/RConn1 -- a/RConn1
  b/RConn1 -- Ideal Switch B/RConn1
  c/RConn1 -- Ideal Switch C/RConn1

== system SPGF_FSK_0000_R2022b/Feed/Q/meas ==
  Add : Sum  Inputs=+++
  GainI : Gain
  GainI0 : Gain
  I A: : spsCurrentMeasurementLib/Current Measurement  PhasorSimulation=off  OutputType=Complex  PSBequivalent=0
  I B: : spsCurrentMeasurementLib/Current Measurement  PhasorSimulation=off  OutputType=Complex  PSBequivalent=0
  I C: : spsCurrentMeasurementLib/Current Measurement  PhasorSimulation=off  OutputType=Complex  PSBequivalent=0
  Mux : Mux  Inputs=3
  A : PMIOPort  Side=Left
  B : PMIOPort  Port=2  Side=Left
  C : PMIOPort  Port=3  Side=Left
  a : PMIOPort  Port=4  Side=Right
  b : PMIOPort  Port=5  Side=Right
  c : PMIOPort  Port=6  Side=Right
  tag scope: CT3I0_F=global, CTIabc_F=global
  wires:
  Mux/1 -> GainI/1
  GainI0/1 -> [CT3I0_F]
  Add/1 -> GainI0/1
  I C:/1 -> Add/3, Mux/3
  I B:/1 -> Add/2, Mux/2
  I A:/1 -> Add/1, Mux/1
  GainI/1 -> [CTIabc_F]
  connections:
  I B:/LConn1 -- B/RConn1
  I C:/LConn1 -- C/RConn1
  I A:/LConn1 -- A/RConn1
  a/RConn1 -- I A:/RConn1
  I B:/RConn1 -- b/RConn1
  I C:/RConn1 -- c/RConn1

== system SPGF_FSK_0000_R2022b/Feed/Q/shunt ==
  A : PMIOPort  Side=Left
  B : PMIOPort  Port=2  Side=Left
  C : PMIOPort  Port=3  Side=Left
  a : PMIOPort  Port=4  Side=Right
  b : PMIOPort  Port=5  Side=Right
  c : PMIOPort  Port=6  Side=Right
  connections:
  C/RConn1 -- c/RConn1
  B/RConn1 -- b/RConn1
  A/RConn1 -- a/RConn1

== system SPGF_FSK_0000_R2022b/Harmonic U/harmonic/Subsystem ==
  clock : Inport
  phase : Inport  Port=2
  Add : Sum
  Add1 : Sum
  Constant1 : Constant  Value=HN
  Constant2 : Constant  Value=Percent./100
  Constant3 : Constant  Value=PhaseH
  Dot Product : DotProduct  OutDataTypeStr=double  RndMeth=Nearest
  Product15 : Product
  Trigonometric Function : Trigonometry  Operator=cos
  amp : Gain  Gain=Voltage*sqrt(2)
  deg2rad : Gain  Gain=pi/180
  omega1 : Gain  Gain=2*pi*Frequency
  o : Outport
  wires:
  Constant3/1 -> Add1/1
  Product15/1 -> Add/1
  deg2rad/1 -> Add/2
  phase/1 -> Add1/2
  Dot Product/1 -> o/1
  Add/1 -> Trigonometric Function/1
  Trigonometric Function/1 -> Dot Product/2
  clock/1 -> Product15/2
  Constant1/1 -> omega1/1
  Add1/1 -> deg2rad/1
  Constant2/1 -> amp/1
  amp/1 -> Dot Product/1
  omega1/1 -> Product15/1

== system SPGF_FSK_0000_R2022b/Harmonic U/harmonic/Subsystem1 ==
  clock : Inport
  phase : Inport  Port=2
  Add : Sum
  Add1 : Sum
  Constant1 : Constant  Value=HN
  Constant2 : Constant  Value=Percent./100
  Constant3 : Constant  Value=PhaseH
  Dot Product : DotProduct  OutDataTypeStr=double  RndMeth=Nearest
  Product15 : Product
  Trigonometric Function : Trigonometry  Operator=cos
  amp : Gain  Gain=Voltage*sqrt(2)
  deg2rad : Gain  Gain=pi/180
  omega1 : Gain  Gain=2*pi*Frequency
  o : Outport
  wires:
  omega1/1 -> Product15/1
  amp/1 -> Dot Product/1
  Constant2/1 -> amp/1
  Add1/1 -> deg2rad/1
  Constant1/1 -> omega1/1
  clock/1 -> Product15/2
  Trigonometric Function/1 -> Dot Product/2
  Add/1 -> Trigonometric Function/1
  Dot Product/1 -> o/1
  phase/1 -> Add1/2
  deg2rad/1 -> Add/2
  Product15/1 -> Add/1
  Constant3/1 -> Add1/1

== system SPGF_FSK_0000_R2022b/Harmonic U/harmonic/Subsystem2 ==
  clock : Inport
  phase : Inport  Port=2
  Add : Sum
  Add1 : Sum
  Constant1 : Constant  Value=HN
  Constant2 : Constant  Value=Percent./100
  Constant3 : Constant  Value=PhaseH
  Dot Product : DotProduct  OutDataTypeStr=double  RndMeth=Nearest
  Product15 : Product
  Trigonometric Function : Trigonometry  Operator=cos
  amp : Gain  Gain=Voltage*sqrt(2)
  deg2rad : Gain  Gain=pi/180
  omega1 : Gain  Gain=2*pi*Frequency
  o : Outport
  wires:
  Constant3/1 -> Add1/1
  Product15/1 -> Add/1
  deg2rad/1 -> Add/2
  phase/1 -> Add1/2
  Dot Product/1 -> o/1
  Add/1 -> Trigonometric Function/1
  Trigonometric Function/1 -> Dot Product/2
  clock/1 -> Product15/2
  Constant1/1 -> omega1/1
  Add1/1 -> deg2rad/1
  Constant2/1 -> amp/1
  amp/1 -> Dot Product/1
  omega1/1 -> Product15/1

== system SPGF_FSK_0000_R2022b/K1/fault/Arcing ==
  m : Inport
  Inter : Inport  Port=2
  Enable : EnablePort  StatesWhenEnabling=reset
  Abs3 : Abs  SaturateOnIntegerOverflow=off
  ArcStrV : Subsystem
  Bistable : spsBistableLib/Bistable  Qpriority=Set  ic=0  Ts=0
      settings: LibrarySourceBlock=sps_lib/Control/Bistable
  Constant1 : Constant  Value=TheoryOfArc
  Constant4 : Constant  Value=TheoryOfArc
  DTC_B : DataTypeConversion  OutDataTypeStr=boolean  SaturateOnIntegerOverflow=off  RndMeth=Floor
  DTC_D : DataTypeConversion  OutDataTypeStr=double  SaturateOnIntegerOverflow=off  RndMeth=Floor
  Demux : Demux  Outputs=2
  Fault A10 : Constant
  Fault A11 : Constant  Value=0
  Peters & Slepian : Subsystem
  Product : Product
  Relational Operator4 : RelationalOperator  OutDataTypeStr=boolean  InputSameDT=off
  SW_1 : MultiPortSwitch  DataPortForDefault=Additional data port  SaturateOnIntegerOverflow=off  InputSameDT=off
  SW_2 : Switch  Criteria=u2 > Threshold  Threshold=2  SaturateOnIntegerOverflow=off  InputSameDT=off
  Subsystem : Subsystem
  Terminator3 : Terminator
  Zero Crossing : Subsystem
  O : Outport  InitialOutput=[0]
  wires:
  Subsystem/1(O) -> Product/2
  Inter/1 -> [Inter]
  Relational Operator4/1 -> Product/1
  [Inter] -> Subsystem/1(I)
  Peters & Slepian/1(O) -> SW_2/1
  [I] -> Peters & Slepian/3(I)
  [Arc] -> Peters & Slepian/2(Arc)
  [I] -> Zero Crossing/1(I)
  Zero Crossing/1(O) -> SW_2/3, Peters & Slepian/1(ZC)  "Petersen"
  ArcStrV/1(Vset) -> Relational Operator4/2
  m/1 -> Demux/1
  Demux/2 -> [V]
  Demux/1 -> [I]
  Constant4/1 -> SW_2/2
  SW_2/1 -> DTC_B/1
  Abs3/1 -> Relational Operator4/1
  [V] -> Abs3/1
  DTC_D/1 -> SW_1/4, SW_1/3
  DTC_B/1 -> Bistable/2
  Bistable/2 -> Terminator3/1
  Product/1 -> [Arc], Bistable/1
  Bistable/1 -> DTC_D/1
  Fault A11/1 -> SW_1/5
  Fault A10/1 -> SW_1/2
  SW_1/1 -> O/1
  Constant1/1 -> SW_1/1

== system SPGF_FSK_0000_R2022b/K1/fault/Count Limiter ==
  I : Inport
  Counter : Subsystem  TreatAsAtomicUnit=on
  Fault A13 : Constant  Value=0
  Fault A3 : Constant
  Switch4 : Switch  Threshold=ArcingNumber  SaturateOnIntegerOverflow=off  InputSameDT=off
  Count : Outport
  O : Outport  Port=2
  wires:
  Counter/1(O) -> Count/1, Switch4/2
  Fault A13/1 -> Switch4/1
  Fault A3/1 -> Counter/1(I)
  I/1 -> Counter/Trigger, Switch4/3
  Switch4/1 -> O/1

== system SPGF_FSK_0000_R2022b/K1/fault/InitialPhaseCtrl ==
  m : Inport
  Enable : EnablePort  StatesWhenEnabling=reset
  Bistable : spsBistableLib/Bistable  Qpriority=Set  ic=0  Ts=0
      settings: LibrarySourceBlock=sps_lib/Control/Bistable
  Bistable1 : spsBistableLib/Bistable  Qpriority=Set  ic=0  Ts=0
      settings: LibrarySourceBlock=sps_lib/Control/Bistable
  Compare To Zero : simulink/Logic and Bit Operations/Compare To Zero  relop=~=  OutDataTypeStr=boolean
  Constant1 : Constant  Value=InitialPhaseCtrl
  DTC_D : DataTypeConversion  OutDataTypeStr=double  SaturateOnIntegerOverflow=off  RndMeth=Floor
  DTC_D1 : DataTypeConversion  OutDataTypeStr=double  SaturateOnIntegerOverflow=off  RndMeth=Floor
  DTC_D2 : DataTypeConversion  OutDataTypeStr=double  SaturateOnIntegerOverflow=off  RndMeth=Floor
  Demux : Demux  Outputs=2
  Fault A11 : Constant
  Hit Crossing : HitCross
  Off Delay : spsOffDelayLib/Off Delay  DelayType=On delay  delay=FaultDelay  ic=0  Ts=0
      settings: LibrarySourceBlock=sps_lib/Control/Off Delay
  Product1 : Product
  SW_1 : MultiPortSwitch  Inputs=2  SaturateOnIntegerOverflow=off  InputSameDT=off
  Terminator : Terminator
  Terminator1 : Terminator
  Terminator3 : Terminator
  O : Outport  InitialOutput=[0]
  wires:
  Bistable1/2 -> Terminator1/1
  DTC_D1/1 -> Product1/2
  Bistable1/1 -> DTC_D1/1
  DTC_D/1 -> SW_1/2
  Fault A11/1 -> SW_1/3
  Off Delay/1 -> Bistable/1
  Bistable/1 -> DTC_D/1
  Bistable/2 -> Terminator3/1
  Constant1/1 -> SW_1/1
  SW_1/1 -> O/1
  Demux/1 -> Terminator/1
  Demux/2 -> [V]
  m/1 -> Demux/1
  Product1/1 -> Off Delay/1
  [V] -> Hit Crossing/1, Compare To Zero/1
  Compare To Zero/1 -> DTC_D2/1
  Hit Crossing/1 -> Bistable1/1
  DTC_D2/1 -> Product1/1

== system SPGF_FSK_0000_R2022b/K1/fault/Interruption ==
  Band-Limited White Noise1 : simulink/Sources/Band-Limited White Noise  Cov=[.1]  Ts=NoiseSampleTime  seed=NoiseSeed
  Constant1 : Constant  Value=TypeOfPause
  Fault A10 : Constant
  Fault A11 : Constant  Value=0
  Multiport Switch : MultiPortSwitch  Inputs=4  DataPortForDefault=Additional data port  SaturateOnIntegerOverflow=off  InputSameDT=off
  Pulse Generator : DiscretePulseGenerator  PulseType=Time based  Period=PulsePeriod  PulseWidth=PulseWidth  PhaseDelay=PhaseDelay
  Rate Transition1 : RateTransition
  Saturation1 : Saturate  UpperLimit=1  LowerLimit=0
  Sign1 : Signum
  "Stair Generator " : spsStairGeneratorLib/Stair Generator  t=SwitchTimes  e=SwitchStatus  Ts=0
  O : Outport
  wires:
  Band-Limited White Noise1/1 -> Sign1/1
  "Stair Generator "/1 -> Multiport Switch/5
  Rate Transition1/1 -> Multiport Switch/3
  Saturation1/1 -> Rate Transition1/1
  Pulse Generator/1 -> Multiport Switch/4
  Constant1/1 -> Multiport Switch/1
  Sign1/1 -> Saturation1/1
  Fault A11/1 -> Multiport Switch/6
  Fault A10/1 -> Multiport Switch/2
  Multiport Switch/1 -> O/1

== system SPGF_FSK_0000_R2022b/K1/fault/Time Delay ==
  Count : Inport
  Control : Inport  Port=2
  Constant1 : Constant  Value=TimeDelay
  Constant3 : Constant  Value=0
  Memory : Memory
  SC_Time5 : Subsystem
      mask Display: disp('Delay');
  SW_Num : Switch  Threshold=ArcingNumber  SaturateOnIntegerOverflow=off  InputSameDT=off
  Selector : Selector  IndexMode=Zero-based  InputPortWidth=ArcingNumber  IndexOptions=Index vector (port)  Indices=[1 4]  OutputSizes=1
  O : Outport
  wires:
  Memory/1 -> SW_Num/3
  Control/1 -> SC_Time5/1(Control)
  SC_Time5/1(Out) -> O/1
  Count/1 -> SW_Num/2, Memory/1
  Constant1/1 -> Selector/1
  Selector/1 -> SC_Time5/2(TimeDelay)
  Constant3/1 -> SW_Num/1
  SW_Num/1 -> Selector/2
